simulink model "lab_Task2"  (R2017b)
settings: Solver=VariableStepAuto  StartTime=0.0  StopTime=10.0  RelTol=1e-3
libraries: simulink x1
settings Model: Creator=ArsalanBangash  LastModifiedBy=ArsalanBangash

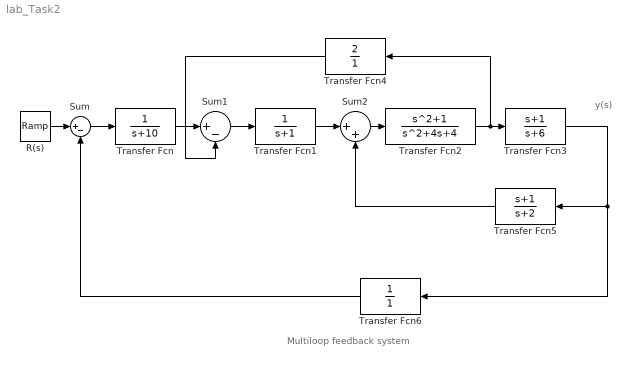
== system lab_Task2 ==
  note: Multiloop feedback system
  note: y(s)
  R(s) : simulink/Sources/Ramp  slope=5  start=0  X0=0
  Sum : Sum  Inputs=|+-
  Sum1 : Sum  Inputs=|+-
  Sum2 : Sum  Inputs=|++
  Transfer Fcn : TransferFcn  Denominator=[1 10]
  Transfer Fcn1 : TransferFcn  Denominator=[1 1]
  Transfer Fcn2 : TransferFcn  Numerator=[1 0 1]  Denominator=[1 4 4]
  Transfer Fcn3 : TransferFcn  Numerator=[1 1]  Denominator=[1 6]
  Transfer Fcn4 : TransferFcn  Numerator=[2]  Denominator=[1]
  Transfer Fcn5 : TransferFcn  Numerator=[1 1]  Denominator=[1 2]
  Transfer Fcn6 : TransferFcn  Denominator=[1]
  wires:
  Sum/1 -> Transfer Fcn/1
  Transfer Fcn/1 -> Sum1/1
  Sum1/1 -> Transfer Fcn1/1
  Transfer Fcn1/1 -> Sum2/1
  Sum2/1 -> Transfer Fcn2/1
  Transfer Fcn2/1 -> Transfer Fcn3/1, Transfer Fcn4/1
  Transfer Fcn4/1 -> Sum1/2
  Transfer Fcn3/1 -> Transfer Fcn6/1, Transfer Fcn5/1
  Transfer Fcn5/1 -> Sum2/2
  Transfer Fcn6/1 -> Sum/2
  R(s)/1 -> Sum/1
